simulink model "untitled11"  (R2023b)
settings: Solver=VariableStepAuto  StartTime=0.0  StopTime=3000  RelTol=1e-3
values from neighbouring files (symbols this model uses):
  final_value = 150    [test.m]
  Hp = Kp /( Tp *s  +1)    [test.m]
  Hpi = Hee * Hp2    [test.m]
  Hr = Hd/ Hf    [test.m]
  Hri = Hdi/Hp2    [test.m]
  initial_value = 25    [test.m]
  step_time = 10    [test.m]
settings Model: Creator=wombelbat  LastModifiedBy=wombelbat

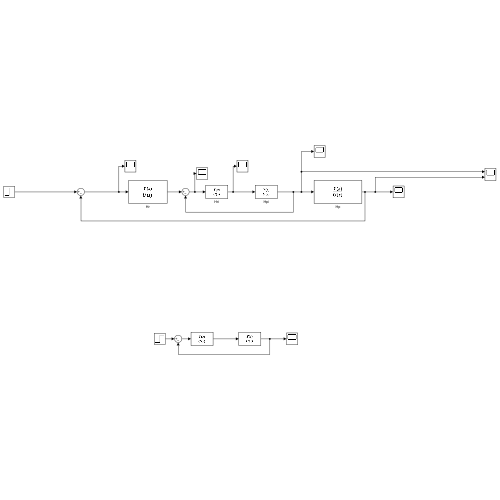
[thumbnail: Simulink's stored preview of the top-level diagram]
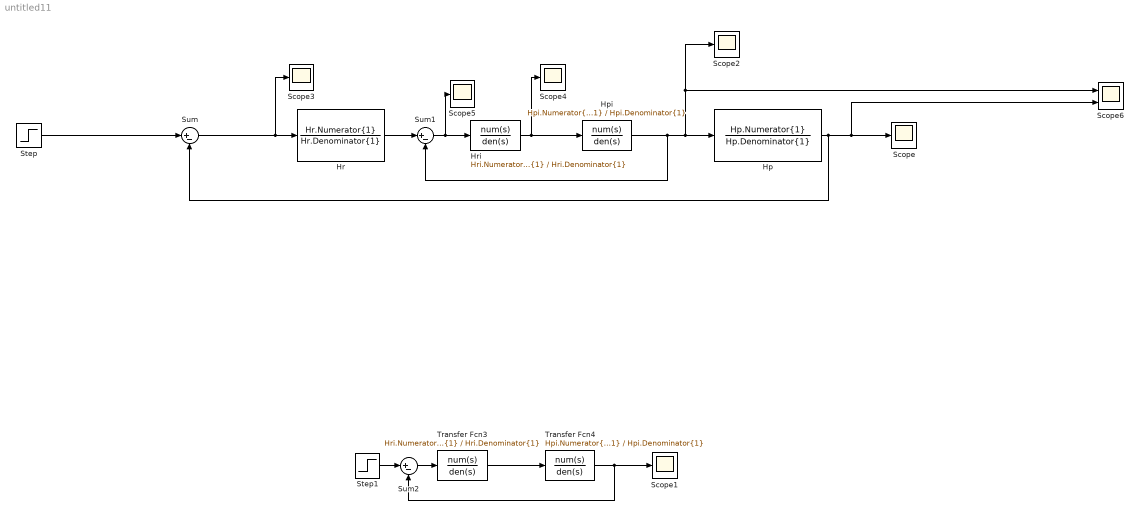
== system untitled11 ==
  Hp : TransferFcn  Numerator=Hp.Numerator{1}  Denominator=Hp.Denominator{1}
  Hpi : TransferFcn  Numerator=Hpi.Numerator{1}  Denominator=Hpi.Denominator{1}
  Hr : TransferFcn  Numerator=Hr.Numerator{1}  Denominator=Hr.Denominator{1}
  Hri : TransferFcn  Numerator=Hri.Numerator{1}  Denominator=Hri.Denominator{1}
  Scope{,1..5} (6 alike) : Scope
  Scope6 : Scope  NumInputPorts=2
  Step : Step  Time=step_time  Before=initial_value  After=final_value  SampleTime=0
  Step1 : Step  Time=step_time  Before=initial_value  After=final_value  SampleTime=0
  Sum : Sum  Inputs=|+-
  Sum1 : Sum  Inputs=|+-
  Sum2 : Sum  Inputs=|+-
  Transfer Fcn3 : TransferFcn  Numerator=Hri.Numerator{1}  Denominator=Hri.Denominator{1}
  Transfer Fcn4 : TransferFcn  Numerator=Hpi.Numerator{1}  Denominator=Hpi.Denominator{1}
  wires:
  Hp/1 -> Sum/2, Scope6/2, Scope/1
  Step/1 -> Sum/1
  Sum/1 -> Scope3/1, Hr/1
  Hpi/1 -> Scope2/1, Scope6/1, Hp/1, Sum1/2
  Hr/1 -> Sum1/1
  Sum1/1 -> Scope5/1, Hri/1
  Sum2/1 -> Transfer Fcn3/1
  Step1/1 -> Sum2/1
  Transfer Fcn3/1 -> Transfer Fcn4/1
  Transfer Fcn4/1 -> Scope1/1, Sum2/2
  Hri/1 -> Scope4/1, Hpi/1
